simulink model "ReferencePIDControl"  (R2019b)
settings: Solver=VariableStepAuto  StartTime=0.0  StopTime=10.0  RelTol=1e-3
values from neighbouring files (symbols this model uses):
  b = 3.5077E-6    [Data_Dict.sldd]
  J = 3.2284E-6    [Data_Dict.sldd]
  Ke = 0.0274    [Data_Dict.sldd]
  Kt = 0.0274    [Data_Dict.sldd]
  L = 2.75E-6    [Data_Dict.sldd]
  R = 4.0    [Data_Dict.sldd]
settings Model: DataDictionary=Data_Dict.sldd  Creator=ip  LastModifiedBy=ip
settings DataIOCC: SaveOutput=off  SaveTime=off

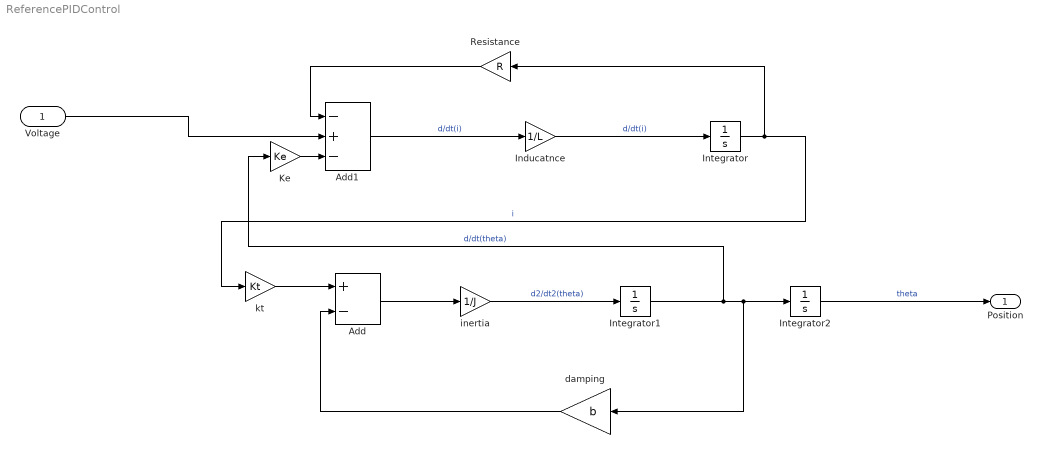
== system ReferencePIDControl ==
  Voltage : Inport  OutDataTypeStr=double  PortDimensions=1  SampleTime=0
  Add : Sum  Inputs=+-
  Add1 : Sum  Inputs=-+-
  Inducatnce : Gain  Gain=1/L
  Integrator : Integrator
  Integrator1 : Integrator
  Integrator2 : Integrator
  Ke : Gain  Gain=Ke
  Resistance : Gain  Gain=R
  damping : Gain  Gain=b
  inertia : Gain  Gain=1/J
  kt : Gain  Gain=Kt
  Position : Outport  OutDataTypeStr=double  PortDimensions=1  SampleTime=0
  wires:
  kt/1 -> Add/1
  Resistance/1 -> Add1/1
  Inducatnce/1 -> Integrator/1  "d/dt(i)"
  Ke/1 -> Add1/3
  inertia/1 -> Integrator1/1  "d2/dt2(theta)"
  damping/1 -> Add/2
  Add1/1 -> Inducatnce/1  "d/dt(i)"
  Add/1 -> inertia/1
  Integrator2/1 -> Position/1  "theta"
  Integrator1/1 -> Integrator2/1, damping/1, Ke/1  "d/dt(theta)"
  Integrator/1 -> Resistance/1, kt/1  "i"
  Voltage/1 -> Add1/2
